simulink model "Piezo"  (R2014b)
settings: Solver=ode4  StartTime=0.0  StopTime=4  FixedStep=1e-4  RelTol=1e-3
libraries: simulink x5
settings Model: Creator=e27269  LastModifiedBy=e27269

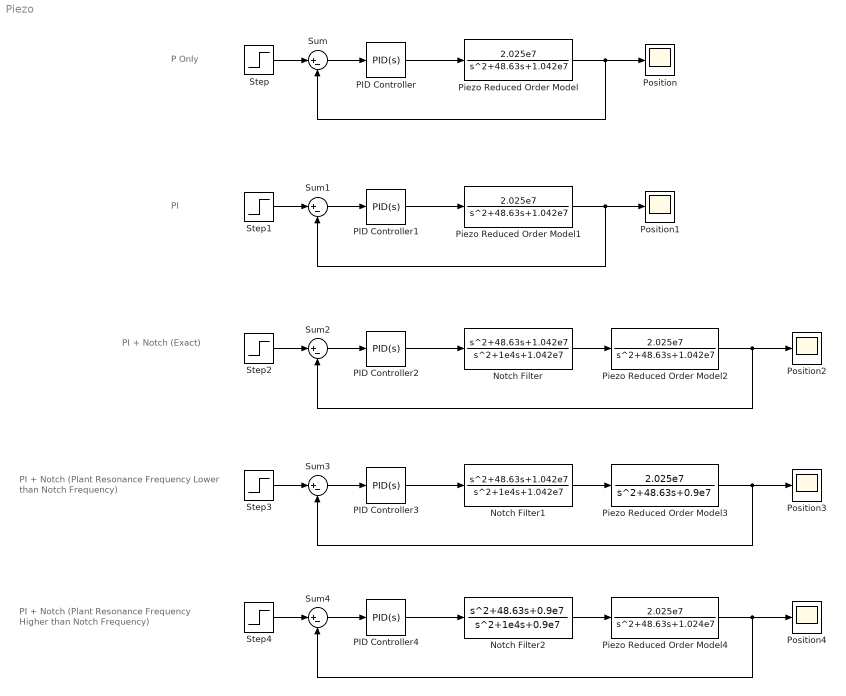
== system Piezo ==
  note: P Only
  note: PI
  note: PI + Notch (Exact)
  note: PI + Notch (Plant Resonance Frequency
      | Lower than Notch Frequency)
  note: PI + Notch (Plant Resonance Frequency
      | Higher than Notch Frequency)
  Notch Filter : TransferFcn  Numerator=[1 48.63 1.042e7]  Denominator=[1 1e4 1.042e7]
  Notch Filter1 : TransferFcn  Numerator=[1 48.63 1.042e7]  Denominator=[1 1e4 1.042e7]
  Notch Filter2 : TransferFcn  Numerator=[1 48.63 0.9e7]  Denominator=[1 1e4 0.9e7]
  PID Controller : simulink/Continuous/PID Controller  Controller=PID  TimeDomain=Continuous-time  SampleTime=-1  IntegratorMethod=Forward Euler  FilterMethod=Forward Euler  Form=Parallel  P=1  I=0  D=0  N=100  InitialConditionSource=internal  InitialConditionForIntegrator=0  InitialConditionForFilter=0  ExternalReset=none  LimitOutput=off  UpperSaturationLimit=inf  LowerSaturationLimit=-inf  LinearizeAsGain=on  AntiWindupMode=none  Kb=1  TrackingMode=off  Kt=1  PParamMin=[]  PParamMax=[]  IParamMin=[]  IParamMax=[]  DParamMin=[]  DParamMax=[]  NParamMin=[]  NParamMax=[]  KbParamMin=[]  KbParamMax=[]  KtParamMin=[]  KtParamMax=[]  POutMin=[]  POutMax=[]  IOutMin=[]  IOutMax=[]  DOutMin=[]  DOutMax=[]  NOutMin=[]  NOutMax=[]  KbOutMin=[]  KbOutMax=[]  KtOutMin=[]  KtOutMax=[]  IntegratorOutMin=[]  IntegratorOutMax=[]  FilterOutMin=[]  FilterOutMax=[]  SumOutMin=[]  SumOutMax=[]  SumI1OutMin=[]  SumI1OutMax=[]  SumI2OutMin=[]  SumI2OutMax=[]  SumI3OutMin=[]  SumI3OutMax=[]  SumDOutMin=[]  SumDOutMax=[]  SaturationOutMin=[]  SaturationOutMax=[]  IntegratorContinuousStateAttributes=''  IntegratorStateMustResolveToSignalObject=off  IntegratorRTWStateStorageClass=Auto  FilterContinuousStateAttributes=''  FilterStateMustResolveToSignalObject=off  FilterRTWStateStorageClass=Auto  DifferentiatorICPrevScaledInput=0  DifferentiatorOutMin=[]  DifferentiatorOutMax=[]  UseFilter=on
  PID Controller{1..4} (4 alike) : simulink/Continuous/PID Controller  Controller=PID  TimeDomain=Continuous-time  SampleTime=-1  IntegratorMethod=Forward Euler  FilterMethod=Forward Euler  Form=Parallel  P=1  I=20  D=0  N=100  InitialConditionSource=internal  InitialConditionForIntegrator=0  InitialConditionForFilter=0  ExternalReset=none  LimitOutput=off  UpperSaturationLimit=inf  LowerSaturationLimit=-inf  LinearizeAsGain=on  AntiWindupMode=none  Kb=1  TrackingMode=off  Kt=1  PParamMin=[]  PParamMax=[]  IParamMin=[]  IParamMax=[]  DParamMin=[]  DParamMax=[]  NParamMin=[]  NParamMax=[]  KbParamMin=[]  KbParamMax=[]  KtParamMin=[]  KtParamMax=[]  POutMin=[]  POutMax=[]  IOutMin=[]  IOutMax=[]  DOutMin=[]  DOutMax=[]  NOutMin=[]  NOutMax=[]  KbOutMin=[]  KbOutMax=[]  KtOutMin=[]  KtOutMax=[]  IntegratorOutMin=[]  IntegratorOutMax=[]  FilterOutMin=[]  FilterOutMax=[]  SumOutMin=[]  SumOutMax=[]  SumI1OutMin=[]  SumI1OutMax=[]  SumI2OutMin=[]  SumI2OutMax=[]  SumI3OutMin=[]  SumI3OutMax=[]  SumDOutMin=[]  SumDOutMax=[]  SaturationOutMin=[]  SaturationOutMax=[]  IntegratorContinuousStateAttributes=''  IntegratorStateMustResolveToSignalObject=off  IntegratorRTWStateStorageClass=Auto  FilterContinuousStateAttributes=''  FilterStateMustResolveToSignalObject=off  FilterRTWStateStorageClass=Auto  DifferentiatorICPrevScaledInput=0  DifferentiatorOutMin=[]  DifferentiatorOutMax=[]  UseFilter=on
  Piezo Reduced Order Model : TransferFcn  Numerator=[2.025e7]  Denominator=[1 48.63 1.042e7]
  Piezo Reduced Order Model1 : TransferFcn  Numerator=[2.025e7]  Denominator=[1 48.63 1.042e7]
  Piezo Reduced Order Model2 : TransferFcn  Numerator=[2.025e7]  Denominator=[1 48.63 1.042e7]
  Piezo Reduced Order Model3 : TransferFcn  Numerator=[2.025e7]  Denominator=[1 48.63 0.9e7]
  Piezo Reduced Order Model4 : TransferFcn  Numerator=[2.025e7]  Denominator=[1 48.63 1.024e7]
  Position{,1..4} (5 alike) : Scope
      Position2 settings: SaveName=ScopeData2
      Position3 settings: SaveName=ScopeData3
      Position4 settings: SaveName=ScopeData4
  Step{,1..4} (5 alike) : Step  SampleTime=0
  Sum{,1..4} (5 alike) : Sum  Inputs=|+-
  wires:
  PID Controller/1 -> Piezo Reduced Order Model/1
  Step/1 -> Sum/1
  Sum/1 -> PID Controller/1
  Piezo Reduced Order Model/1 -> Position/1, Sum/2
  PID Controller1/1 -> Piezo Reduced Order Model1/1
  Step1/1 -> Sum1/1
  Sum1/1 -> PID Controller1/1
  Piezo Reduced Order Model1/1 -> Position1/1, Sum1/2
  Step2/1 -> Sum2/1
  Sum2/1 -> PID Controller2/1
  Piezo Reduced Order Model2/1 -> Sum2/2, Position2/1
  Notch Filter/1 -> Piezo Reduced Order Model2/1
  PID Controller2/1 -> Notch Filter/1
  Step3/1 -> Sum3/1
  Sum3/1 -> PID Controller3/1
  Piezo Reduced Order Model3/1 -> Sum3/2, Position3/1
  Notch Filter1/1 -> Piezo Reduced Order Model3/1
  PID Controller3/1 -> Notch Filter1/1
  Step4/1 -> Sum4/1
  Sum4/1 -> PID Controller4/1
  Piezo Reduced Order Model4/1 -> Sum4/2, Position4/1
  Notch Filter2/1 -> Piezo Reduced Order Model4/1
  PID Controller4/1 -> Notch Filter2/1
